simulink model "model5_power"  (R2019b)
settings: Solver=VariableStepAuto  StartTime=0.0  StopTime=15*3600  RelTol=1e-3
PreLoadFcn:
  | % Set physical parameters
  | panelMotorParams;
  | 
  | % Load sun position data for tracking
  | load sunPositionData;
values from neighbouring files (symbols this model uses):
  A = w*l    (= 1.456)    [panelMotorParams.m]
  beta = pi/4    (= 0.785398163397)    [panelMotorParams.m]
  J = m/12*(l^2*cos(beta)^2+d^2*sin(beta)^2+w^2)    [panelMotorParams.m]
  Kd = 5    [panelMotorParams.m]
  Kf = 0.07    [panelMotorParams.m]
  Kg = 2000    [panelMotorParams.m]
  Kt = 0.07    [panelMotorParams.m]
  L = 1e-5    (= 1e-05)    [panelMotorParams.m]
  R = 10    [panelMotorParams.m]
libraries: simulink x1
settings Model: Creator=bneiswan  LastModifiedBy=bneiswan
settings DataIOCC: ExternalInput=[sunTime,sunPosition,sunElevation]  LoadExternalInput=on

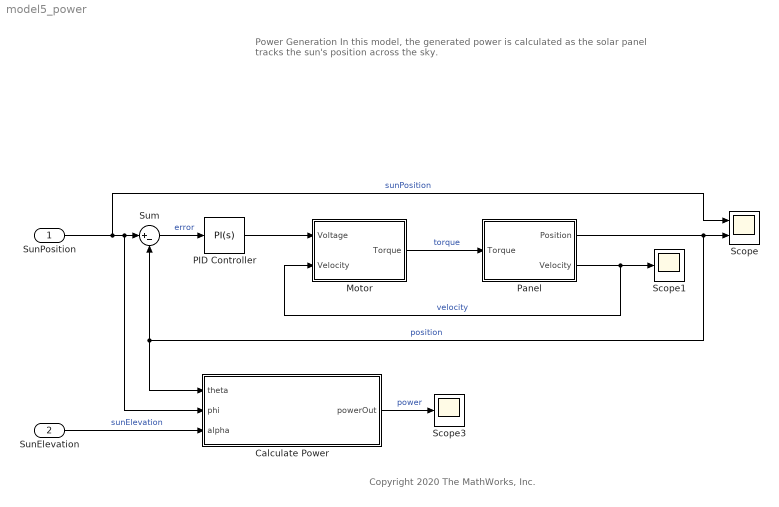
== system model5_power ==
  note: Copyright 2020 The MathWorks, Inc.
  note: Power Generation
      |
      | In this model, the generated power is calculated as the solar panel tracks the sun's position across the sky.
  SunPosition : Inport
  SunElevation : Inport  Port=2
  Calculate Power : MATLAB Function  TreatAsAtomicUnit=on
  Motor : Subsystem
  PID Controller : simulink/Continuous/PID Controller  Controller=PI  Form=Parallel  TimeDomain=Continuous-time  SampleTime=-1  IntegratorMethod=Forward Euler  FilterMethod=Forward Euler  ControllerParametersSource=internal  P=240  I=180  D=0  UseFilter=on  N=100  TunerSelectOption=Transfer Function Based (PID Tuner App)  InitialConditionSource=internal  InitialConditionForIntegrator=0  InitialConditionForFilter=0  DifferentiatorICPrevScaledInput=0  ExternalReset=none  TrackingMode=off  Kt=1  LimitOutput=off  UpperSaturationLimit=inf  LowerSaturationLimit=-inf  LinearizeAsGain=on  AntiWindupMode=none  Kb=1  POutMin=[]  POutMax=[]  IOutMin=[]  IOutMax=[]  DOutMin=[]  DOutMax=[]  NOutMin=[]  NOutMax=[]  SumOutMin=[]  SumOutMax=[]  SaturationOutMin=[]  SaturationOutMax=[]  PParamMin=[]  PParamMax=[]  IParamMin=[]  IParamMax=[]  DParamMin=[]  DParamMax=[]  NParamMin=[]  NParamMax=[]  KbParamMin=[]  KbParamMax=[]  KtParamMin=[]  KtParamMax=[]  KbOutMin=[]  KbOutMax=[]  KtOutMin=[]  KtOutMax=[]  IntegratorOutMin=[]  IntegratorOutMax=[]  FilterOutMin=[]  FilterOutMax=[]  SumI1OutMin=[]  SumI1OutMax=[]  SumI2OutMin=[]  SumI2OutMax=[]  SumI3OutMin=[]  SumI3OutMax=[]  SumI4OutMin=[]  SumI4OutMax=[]  SumDOutMin=[]  SumDOutMax=[]  DifferentiatorOutMin=[]  DifferentiatorOutMax=[]  FilterDiffOutCoefMin=[]  FilterDiffOutCoefMax=[]  ReciprocalOutMin=[]  ReciprocalOutMax=[]  SumDenOutMin=[]  SumDenOutMax=[]  SumNumOutMin=[]  SumNumOutMax=[]  DivideOutMin=[]  DivideOutMax=[]  IntegratorContinuousStateAttributes=''  IntegratorStateMustResolveToSignalObject=off  IntegratorRTWStateStorageClass=Auto  FilterContinuousStateAttributes=''  FilterStateMustResolveToSignalObject=off  FilterRTWStateStorageClass=Auto  ParallelPVariant=InternalParameters  IdealPVariant=Disabled  IVariant=InternalParameters  DVariant=Disabled  IntegratorVariant=Continuous  SatVariant=Disabled  AWVariant=Passthrough  PCopyVariant=Disabled  TRVariant=Disabled  FdbkBlocksVariant=Forward  IdealPFdbkVariant=Disabled  SatFdbkVariant=Disabled  DerivativeFilterVariant=Disabled  NVariant=Disabled  NCopyVariant=Disabled_SignalSpec  FilterICVariant=Disabled  IntegratorICVariant=InternalICs  ExternalResetVariant=Disabled  TRSumVariant=Passthrough  SumFdbkVariant=Disabled  SumVariant=Sum_PI
  Panel : Subsystem
  Scope : Scope  NumInputPorts=2
  Scope1 : Scope
  Scope3 : Scope
  Sum : Sum  Inputs=|+-
  wires:
  Calculate Power/1(powerOut) -> Scope3/1  "power"
  SunElevation/1 -> Calculate Power/3(alpha)  "sunElevation"
  PID Controller/1 -> Motor/1(Voltage)
  Panel/1(Position) -> Scope/2, Sum/2, Calculate Power/1(theta)  "position"
  SunPosition/1 -> Calculate Power/2(phi), Sum/1, Scope/1  "sunPosition"
  Sum/1 -> PID Controller/1  "error"
  Panel/2(Velocity) -> Motor/2(Velocity), Scope1/1  "velocity"
  Motor/1(Torque) -> Panel/1(Torque)  "torque"

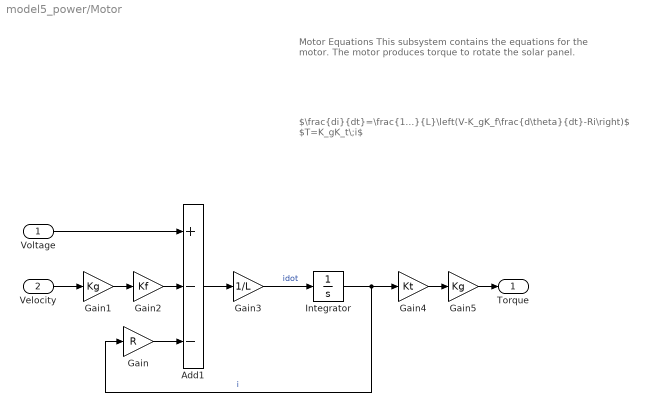
== system model5_power/Motor ==
  note: $\frac{di}{dt}=\frac{1}{L}\left(V-K_gK_f\frac{d\theta}{dt}-Ri\right)$
      | $T=K_gK_t\;i$
  note: Motor Equations
      |
      | This subsystem contains the equations for the motor. The motor produces torque to rotate the solar panel.
  Voltage : Inport
  Velocity : Inport  Port=2
  Add1 : Sum  Inputs=+--
  Gain : Gain  Gain=R
  Gain1 : Gain  Gain=Kg
  Gain2 : Gain  Gain=Kf
  Gain3 : Gain  Gain=1/L
  Gain4 : Gain  Gain=Kt
  Gain5 : Gain  Gain=Kg
  Integrator : Integrator
  Torque : Outport
  wires:
  Voltage/1 -> Add1/1
  Gain2/1 -> Add1/2
  Gain3/1 -> Integrator/1  "idot"
  Gain/1 -> Add1/3
  Integrator/1 -> Gain4/1, Gain/1  "i"
  Add1/1 -> Gain3/1
  Velocity/1 -> Gain1/1
  Gain4/1 -> Gain5/1
  Gain1/1 -> Gain2/1
  Gain5/1 -> Torque/1

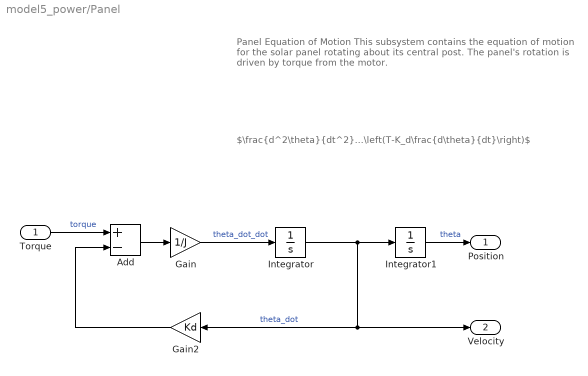
== system model5_power/Panel ==
  note: $\frac{d^2\theta}{dt^2}=\frac{1}{J}\left(T-K_d\frac{d\theta}{dt}\right)$
  note: Panel Equation of Motion
      |
      | This subsystem contains the equation of motion for the solar panel rotating about its central post. The panel's rotation is driven by torque from the motor.
  Torque : Inport
  Add : Sum  Inputs=+-
  Gain : Gain  Gain=1/J
  Gain2 : Gain  Gain=Kd
  Integrator : Integrator
  Integrator1 : Integrator
  Position : Outport
  Velocity : Outport  Port=2
  wires:
  Torque/1 -> Add/1  "torque"
  Add/1 -> Gain/1
  Integrator/1 -> Integrator1/1, Velocity/1, Gain2/1  "theta_dot"
  Gain2/1 -> Add/2
  Gain/1 -> Integrator/1  "theta_dot_dot"
  Integrator1/1 -> Position/1  "theta"

== matlab function model5_power/Calculate Power ==
  data: theta input; phi input; alpha input; powerOut output; A parameter; beta parameter
function powerOut = CalculatePower(theta, phi, alpha, A, beta)

% Calculate dot product of the incident sun and panel normal vectors
dot_prod = sin(beta)*sin(pi/2-alpha)*cos(theta-phi) ...
    + cos(beta)*cos(pi/2-alpha);

% Calculate the direct power
powerOut = 1.353*0.7.^(sin(alpha).^-0.678)*dot_prod*A*0.195*1000; % W

% Replace negative power values with zero (sun is behind the panel)
powerOut = max(powerOut,0);
